simulink model "mobile_gravity_field"  (R2023a)
settings: Solver=VariableStepAuto  StartTime=0.0  StopTime=10.0  RelTol=1e-3
settings Model: Creator=crt4254  LastModifiedBy=crt4254

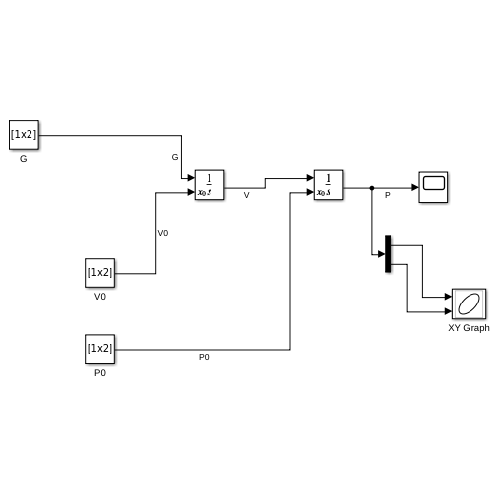
[thumbnail: Simulink's stored preview of the top-level diagram]
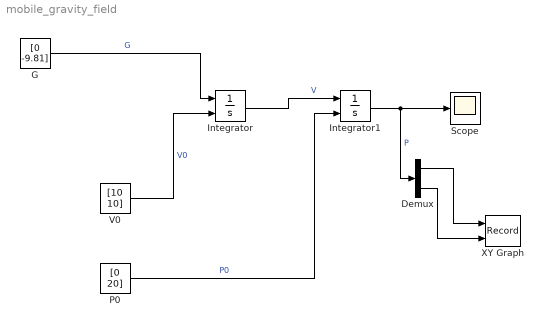
== system mobile_gravity_field ==
  Demux : Demux  Outputs=2
  G : Constant  Value=[0 -9.81]
  Integrator : Integrator  InitialConditionSource=external
  Integrator1 : Integrator  InitialConditionSource=external
  P0 : Constant  Value=[0 20]
  Scope : Scope
  V0 : Constant  Value=[10 10]
  XY Graph : Record  FileSettingsInternal="{\"entries\":[{\"content\":{\"excelSettings\":{\"content\":{},\"type\":\"Streamout.ExcelSettings\"}},\"type\":\"Streamout.FileSettingStorage\",\"uuid\":\"ede03986-e9c2-4f60-99ea-1667be0f6faf\"}],\"packageUris\":[\"http://schema.mathworks.com/mf0/streamout_blocks/R2020a\"],\"version\":\"1.0\"}"  Layout=[1 1]  SignalsInternal="{\"entries\":[{\"content\":{\"signals\":[{\"content\":{\"blockPath\":[\"untitled/XY Graph\"],\"dimensions\":[1],\"domain\":\"untitled/XY Graph\",\"lineColor\":\"#a2142f\",\"plots\":[1],\"port\":1,\"sid\":[\"\"],\"signalID\":59,\"signalName\":\"Demux:1\"},\"type\":\"RecordBlkView.Signal\",\"uuid\":\"53d0e130-440f-454e-b5e6-c81a125c8e8f\"},{\"content\":{\"blockPath\":[\"untitled/XY Graph\"],\"dimensions\":[1],\"domain\":\"untitled/XY Graph\",\"lineColor\":\"#139fff\",\"plots\":[1],\"port\":2,\"sid\":[\"\"],\"signalID\":63,\"signalName\":\"Demux:2\"},\"type\":\"RecordBlkView.Signal\",\"uuid\":\"00c6d273-a940-40bc-a7d6-e615642112d0\"}]},\"type\":\"RecordBlkView.InputSignals\",\"uuid\":\"3c5b9a83-ab1e-4753-8c0c-5eaa88a27892\"}],\"packageUris\":[\"http://schema.mathworks.com/mf0/streamout_blocks/R2020a\"],\"version\":\"1.0\"}"  VisualizationBindings="{\"xyplotplugin\":{\"info\":[{\"series\":[{\"bindingParametersList\":[{\"parameter\":\"X-Axis\",\"signalID\":59,\"signalName\":\"Demux:1\"},{\"parameter\":\"Y-Axis\",\"signalID\":63,\"signalName\":\"Demux:2\"}],\"seriesID\":27050}],\"subplotID\":1}]}}"  CompatibilityTag=XY
  wires:
  G/1 -> Integrator/1  "G"
  V0/1 -> Integrator/2  "V0"
  Integrator/1 -> Integrator1/1  "V"
  P0/1 -> Integrator1/2  "P0"
  Integrator1/1 -> Demux/1, Scope/1  "P"
  Demux/1 -> XY Graph/1
  Demux/2 -> XY Graph/2
